simulink model "untitled"  (R2014a)
settings: Solver=ode45  StartTime=0.0  StopTime=1  RelTol=1e-3
libraries: powerlib x8, powerlib_meascontrol x6
settings Model: Creator=nusrat  LastModifiedBy=nusrat
settings SFSimCC: SimGenImportedTypeDefs=on

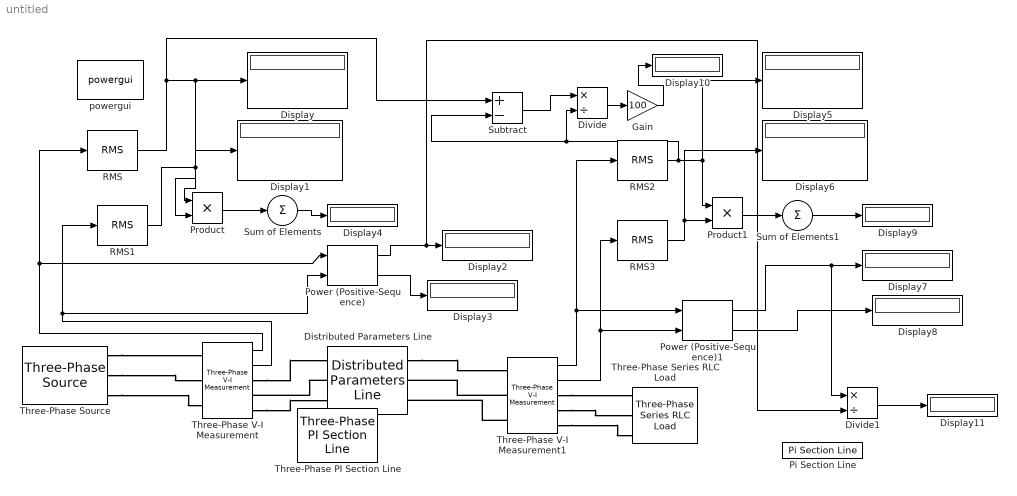
== system untitled ==
  Display{,1..11} (12 alike) : Display
  Distributed Parameters Line : powerlib/Elements/Distributed Parameters Line  Phases=3  Frequency=60  Resistance=[0 0]  Inductance="[0.97e-3  0.97e-3]"  Capacitance=[11.94e-9 11.9e-9]  Length=300  x1=[0 0 0 0; 0.0001244 0 0 0; 0.0002488 0 0 0; 0.0003733 0 0 0; 0.0004977 0 0 0; 0.0006221 0 0 0]  x2=[0 0 0 0; 0.0001244 0 0 0; 0.0002488 0 0 0; 0.0003733 0 0 0; 0.0004977 0 0 0; 0.0006221 0 0 0]  x3=[0 0 0 0; 0.0001244 0 0 0; 0.0002488 0 0 0; 0.0003733 0 0 0; 0.0004977 0 0 0; 0.0006221 0 0 0]  x4=[0 0 0 0; 0.0001244 0 0 0; 0.0002488 0 0 0; 0.0003733 0 0 0; 0.0004977 0 0 0; 0.0006221 0 0 0]  x5=0  V1=[5.821e-11 6.175e+05 6.175e+05;377 377 377;1.187 0.4197 -1.151]  V2=[9.318e-11 5.012e+05 5.012e+05;377 377 377;0.2905 0.1381 -1.433]  I1=[2.357e-13 1213 1213;377 377 377;3.024 1.196 -0.3746]  I2=[4.547e-13 3571 3571;377 377 377;2.757 -0.2055 -1.776]  nHarmo=1  Measurements=None
  Divide : Product  Inputs=*/
  Divide1 : Product  Inputs=*/
  Gain : Gain  Gain=100  SampleTime=0
  Pi Section Line : powerlib/Elements/Pi Section Line  LConnTagsString=__new0  RConnTagsString=__new0  Frequency=60  Resistance=0.01273  Inductance=0.9337e-3  Capacitance=12.74e-9  Length=100  PiSections=1  Measurements=None
      settings: AttributesFormatString=\n
  Power (Positive-Sequence) : powerlib_meascontrol/Measurements/Power (Positive-Sequence)  Freq=60  Vinit=[0, 0]  Iinit=[0, 0]  Ts=0
  Power (Positive-Sequence)1 : powerlib_meascontrol/Measurements/Power (Positive-Sequence)  Freq=60  Vinit=[0, 0]  Iinit=[0, 0]  Ts=0
  Product : Product
  Product1 : Product
  RMS{,1..3} (4 alike) : powerlib_meascontrol/Measurements/RMS  TrueRMS=on  Freq=60  RMSInit=120  Ts=0
  Subtract : Sum  Inputs=+-
  Sum of Elements : Sum  Inputs=+
  Sum of Elements1 : Sum  Inputs=+
  Three-Phase PI Section Line : powerlib/Elements/Three-Phase PI Section Line  LConnTagsString=a|b|c  RConnTagsString=A|B|C  Frequency=60  Resistances=[ 0.01273 0.3864]  Inductances="[ 0.9337e-3  4.1264e-3]"  Capacitances=[12.74e-9 7.751e-9]  Length=100
  Three-Phase Series RLC Load : powerlib/Elements/Three-Phase Series RLC Load  LConnTagsString=A|B|C  Configuration=Y (grounded)  NominalVoltage=500e3  NominalFrequency=60  ActivePower=800e6  InductivePower=600e6  CapacitivePower=0  Measurements=None  LoadType=constant Z
  Three-Phase V-I Measurement : powerlib/Measurements/Three-Phase V-I Measurement  VoltageMeasurement=phase-to-ground  SetLabelV=off  LabelV=Vabc  Vpu=off  VpuLL=off  CurrentMeasurement=yes  SetLabelI=off  LabelI=Iabc  Ipu=off  Pbase=100e6  Vbase=500e3  OutputType=Complex  PhasorSimulation=off  PSBequivalent=0
  Three-Phase V-I Measurement1 : powerlib/Measurements/Three-Phase V-I Measurement  VoltageMeasurement=phase-to-ground  SetLabelV=off  LabelV=Vabc  Vpu=off  VpuLL=off  CurrentMeasurement=yes  SetLabelI=off  LabelI=Iabc  Ipu=off  Pbase=100e6  Vbase=500e3  OutputType=Complex  PhasorSimulation=off  PSBequivalent=0
  Three-Phase Source : powerlib/Electrical Sources/Three-Phase Source  Voltage=617.53e3  PhaseAngle=16.1  Frequency=60  InternalConnection=Yg  SpecifyImpedance=off  Resistance=0  Inductance=0  ShortCircuitLevel=100e6  BaseVoltage=0  XRratio=7  BusType=swing  Pref=0  Qref=0  Qmin=-inf  Qmax=inf
  powergui : powerlib/powergui  Priority=1  SimulationMode=Continuous  SolverType=Tustin  SampleTime=50e-6  frequency=60  SPID=off  DisableSnubberDevices=off  DisableRonSwitches=off  DisableVfSwitches=off  SwTol=0  Interpol=off  DisplayEquations=off  Ts=0  methode=off  frequencyindice=60  Pbase=100e6  ErrMax=1e-4  Iterations=50  UnitsV=kV  UnitsW=MW  FunctionMessages=off  echomessages=off  HookPort=off  EnableUseOfTLC=off  x0status=blocks  RestoreLinks=warning  ResistiveCurrentMeasurement=off  Frange=[0:2:500]  Ylog=off  Xlog=on  ShowGrid=off  save=off  variable=ZData  structure=0  ZoomFFT=off  StartTime=0.0  cycles=1  DisplayStyle=1  fundamental=60  FreqAxis=off  MaxFrequency=1000  frequencyindicesteady=1  RmsSteady=1  display=off
  wires:
  Three-Phase V-I Measurement/1 -> RMS/1, Power (Positive-Sequence)/1
  RMS/1 -> Subtract/1, Product/1, Display/1
  Three-Phase V-I Measurement/2 -> RMS1/1, Power (Positive-Sequence)/2
  RMS1/1 -> Product/2, Display1/1
  Power (Positive-Sequence)/1 -> Divide1/2, Display2/1
  Power (Positive-Sequence)/2 -> Display3/1
  Product/1 -> Sum of Elements/1
  Three-Phase V-I Measurement1/1 -> RMS2/1, Power (Positive-Sequence)1/1
  RMS2/1 -> Divide/2, Subtract/2, Product1/1, Display5/1
  Three-Phase V-I Measurement1/2 -> RMS3/1, Power (Positive-Sequence)1/2
  RMS3/1 -> Display6/1, Product1/2
  Power (Positive-Sequence)1/1 -> Divide1/1, Display7/1
  Power (Positive-Sequence)1/2 -> Display8/1
  Product1/1 -> Sum of Elements1/1
  Sum of Elements1/1 -> Display9/1
  Subtract/1 -> Divide/1
  Divide/1 -> Gain/1
  Gain/1 -> Display10/1
  Sum of Elements/1 -> Display4/1
  Divide1/1 -> Display11/1
  connections:
  Three-Phase Source/RConn1 -- Three-Phase V-I Measurement/LConn1
  Three-Phase Source/RConn2 -- Three-Phase V-I Measurement/LConn2
  Three-Phase Source/RConn3 -- Three-Phase V-I Measurement/LConn3
  Three-Phase V-I Measurement/RConn1 -- Distributed Parameters Line/LConn1
  Distributed Parameters Line/LConn2 -- Three-Phase V-I Measurement/RConn2
  Three-Phase V-I Measurement/RConn3 -- Distributed Parameters Line/LConn3
  Distributed Parameters Line/RConn1 -- Three-Phase V-I Measurement1/LConn1
  Three-Phase V-I Measurement1/LConn2 -- Distributed Parameters Line/RConn2
  Three-Phase V-I Measurement1/LConn3 -- Distributed Parameters Line/RConn3
  Three-Phase V-I Measurement1/RConn1 -- Three-Phase Series RLC Load/LConn1
  Three-Phase V-I Measurement1/RConn2 -- Three-Phase Series RLC Load/LConn2
  Three-Phase V-I Measurement1/RConn3 -- Three-Phase Series RLC Load/LConn3
